simulink model "LAB1"  (R2021a)
settings: Solver=VariableStepAuto  StartTime=0.0  StopTime=10.0  RelTol=1e-3
values from neighbouring files (symbols this model uses):
  a1 = 6    [lab1.m]
  c1 = 4    [lab1.m]
settings Model: Creator=rfier  LastModifiedBy=rfier

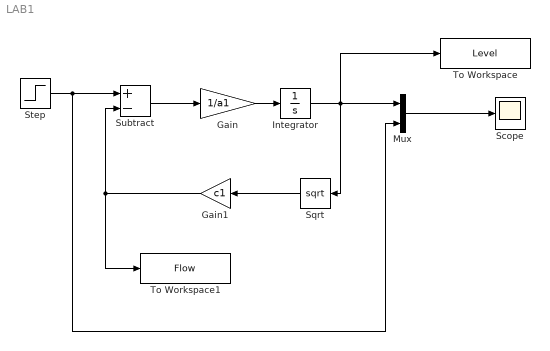
== system LAB1 ==
  Gain : Gain  Gain=1/a1
  Gain1 : Gain  Gain=c1
  Integrator : Integrator
  Mux : Mux  Inputs=2
  Scope : Scope
  Sqrt : Sqrt  SaturateOnIntegerOverflow=on
  Step : Step  SampleTime=0
  Subtract : Sum  Inputs=+-
  To Workspace : ToWorkspace  VariableName=Level  SaveFormat=Timeseries  SampleTime=-1
  To Workspace1 : ToWorkspace  VariableName=Flow  SaveFormat=Timeseries  SampleTime=-1
  wires:
  Gain1/1 -> To Workspace1/1, Subtract/2
  Subtract/1 -> Gain/1
  Gain/1 -> Integrator/1
  Sqrt/1 -> Gain1/1
  Integrator/1 -> Sqrt/1, To Workspace/1, Mux/1
  Mux/1 -> Scope/1
  Step/1 -> Mux/2, Subtract/1
